simulink model "Wall_Model_Version_1_5_2016a"  (R2017b)
settings: Solver=ode3  StartTime=0.0  StopTime=1000  FixedStep=Ts  RelTol=1e-3  EnableMultiTasking=on
InitFcn:
  | clc;
  | clear all;
  | close all;
  | Ts=1
  | Duration=36000;
  | %% Coefficients of Rs and Cs
  | 
  | %% Front Wall
  | l1 = 7.37;
  | b1 = 2.63;
  | y1 = 0.5;
  | x1 = 0.33;
  | y2 = 0.5;
  | x2 = 0.33;
  | x3 = 0.33;
  | 
  | %% Left Wall
  | l2 = 10.11;
  | b2 = 2.63;
  | y3 = 0.5;
  | x4 = 0.33;
  | y4 = 0.5;
  | x5 = 0.33;
  | x6 = 0.33;
  | 
  | %% Left Wall Glass
  | x4_g = 0.5;
  | x5_g = 0.5;
  | y3_g = 1;
  | 
  | %% Right Wall
  | l3 = 7.37;
  | b3 = 2.63;
  | y5 = 0.5;
  | x7 = 0.33;
  | y6 = 0.5;
  | x8 = 0.33;
  | x9 = 0.33;
  | 
  | %% Back Wall
  | l4 = 10.11;
  | b4 = 2.63;
  | y7 = 1;
  | x10 = 0.5;
  | %y8 = 0.5;
  | x11 = 0.5;
  | %x12= 0.33;
  | 
  | %% Roof
  | l5 = 10.11;
  | b5 = 7.37;
  | y9 = 0.5;
  | x13 = 0.33;
  | y10 = 0.5;
  | x14 = 0.33;
  | x15 = 0.33;
  | 
  | %% Floor
  | l6 = 10.11;
  | b6 = 7.37;
  | y11 = 0.5;
  | x16 = 0.33;
  | y12 = 0.5;
  | x17 = 0.33;
  | x18 = 0.33;
  | 
  | %%Areas
  | A1 = l1 * b1;
  | A2 = l2 * b2;
  | A3 = l3 * b3;
  | A4 = l4 * b4;
  | A5 = l5 * b5;
  | A6 = l6 * b6;
  | 
  | %% Initial Temperatures at the surfaces
  | T1_initial_front=301;
  | T2_initial_front=300;
  | 
  | T1_initial_left=301;
  | T2_initial_left=300;
  | 
  | T1_initial_right=301;
  | T2_initial_right=300;
  | 
  | T1_initial_back=301;
  | T2_initial_back=300;
  | 
  | T1_initial_roof=301;
  | T2_initial_roof=300;
  | 
  | T1_initial_floor=301;
  | T2_initial_floor=300;
  | 
  | ri = 0.1300; % m2 K/W resistance of inner surface of brick wall
  | rso = 0.04; % m2 K/W resistance of outer surface of the wall
  | 
  | %% Density of Building materials in the room
  | p_conc    = 1700; % kg/m3 density of concrete
  | p_pstr     = 1000; % kg/m3 density of plastering
  | p_gb       = 1100; % kg/m3 density of gypsum board
  | p_glass    = 2500; % kg/m3 density of glass
  | p_swood  = 550;   % kg/m3 density of soft-wood
  | 
  | %% Thermal heat capacity of the building materials in the room
  | c_conc    = 840;  % J/kg K heat capacity of concrete
  | c_pstr     = 1000;  %J/kg K heat capacity of plastering
  | c_gb       = 1090; % J/kg K heat capacity of gypsum board
  | c_glass    = 840;  % J/kg K heat capacity of glass
  | c_swood  = 1700; % J/kg K heat capacity of soft-wood
  | 
  | %% Thermal conductivity(lamda) of building materials in the room
  | l_conc    = 0.8;  % W/m K Thermal conductivity of concrete
  | l_pstr     = 0.013;  % W/m K Thermal conductivity of plastering
  | l_gb       = 0.35; % W/m K Thermal conductivity of gypsum board
  | l_glass    = 0.8;  % W/m K Thermal conductivity of glass
  | l_swood  = 0.08; % W/m K Thermal conductivity of soft-wood
  | 
  | %% Standard thickness of materials used
  | d_conc = 0.01;  % m Thickness of concrete BCA standard
  | d_pstr = 0.005; % m Thickness of plastering BCA standard
  | d_glass = 0.015; % m Thickness of glass wall widely used
  | d_swood = 0.01; % m Thickness of softwood on the right wall
  | d_gb = 0.015; % m Thickness of gypsum board
  | 
  | %% Resistance and Capacitance of front Wall
  | Rth1 =( ri + rso + (d_conc/l_conc) + (d_pstr/l_pstr))/(A1); % Thermal resistance
  | Cth1 = A1*(d_conc*p_conc*c_conc + d_pstr*p_pstr*c_pstr) ; % Thermal Capacitance
  | 
  | %% Resistance and Capacitance of left Wall concrete
  | A_conc = A2 * 0.5; % Half of the wall on the left is  glass wall
  | Rth2 =( ri + rso + (d_conc/l_conc) + (d_pstr/l_pstr))/(A_conc); % Thermal resistance
  | Cth2 = A_conc*(d_conc*p_conc*c_conc + d_pstr*p_pstr*c_pstr); % Thermal Capacitance
  | 
  | %% Resistance and Capacitance of left Wall glass
  | A_glass = A2 * 0.5; % Half of the wall on the left is  glass wall
  | Rth2_g =(d_glass/l_glass) /(A_glass); % Thermal resistance
  | Cth2_g = A_glass*(d_glass*p_glass*c_glass ); % Thermal Capacitance
  | 
  | %% Resistance and Capacitance of right Wall
  | Rth3 = ( ri + rso+ (d_conc/l_conc) + (d_swood/l_swood))/(A3);% Thermal resistance
  | Cth3 = A3*(d_swood*p_swood*c_swood + d_conc*p_conc*c_conc ); % Thermal Capacitance
  | 
  | %% Resistance and Capacitance of back Wall
  | Rth4 =(d_glass/l_glass) /(A4); % Thermal resistance
  | Cth4 = A4*(d_glass*p_glass*c_glass ); % Thermal Capacitance
  | 
  | %% Resistance and Capacitance of roof Wall
  | Rth5 = (d_gb/l_gb)/(A5);% Thermal resistance
  | Cth5 = A5*(d_gb*p_gb*c_gb ); % Thermal Capacitance
  | 
  | %% Resistance and Capacitance of floor Wall
  | Rth6 = (d_gb/l_gb)/(A6);% Thermal resistance
  | Cth6 = A6*(d_gb*p_gb*c_gb ); % Thermal Capacitance
  | 
  | %% Volume and mass of room
  | density_of_air = 1.184; % kg/m3 at 25 deg. K
  | volume = l1*l2*b1; % m3
  | mass = volume * density_of_air ;% kg
  | specific_heat = 1.005; % J/kg deg.K
  | tic;
libraries: powerlib x69, simulink x1
settings Model: Creator=elekkr  LastModifiedBy=e0154145
settings DataIOCC: LimitDataPoints=on  SaveFormat=Array
settings OptimizationCC: LifeSpan=inf
settings DebuggingCC: UnconnectedInputMsg=none  UnconnectedOutputMsg=none  UnconnectedLineMsg=none  SFUnexpectedBacktrackingDiag=warning  SFNoUnconditionalDefaultTransitionDiag=warning  SFExecutionAtInitializationDiag=none
settings HardwareCC: ProdBitPerPointer=32  ProdBitPerSizeT=32  ProdBitPerPtrDiffT=32  ProdLargestAtomicFloat=None  ProdIntDivRoundTo=Undefined  ProdEndianess=Unspecified  ProdWordSize=32  ProdHWDeviceType=32-bit Generic
settings ModelReferenceCC: PropagateSignalLabelsOutOfModel=off
settings CodeAppCC: StateflowObjectComments=on
settings GRTTargetCC: TargetLangStandard=C89/C90 (ANSI)  GeneratePreprocessorConditionals=Disable all
settings ConfigComp: CovMetricSettings=dw  CovHtmlReporting=on  CovSaveCumulativeToWorkspaceVar=on  CovSaveSingleToWorkspaceVar=on  CovExternalEMLEnable=off
settings SimscapeCC: SimscapeNormalizeSystem=off

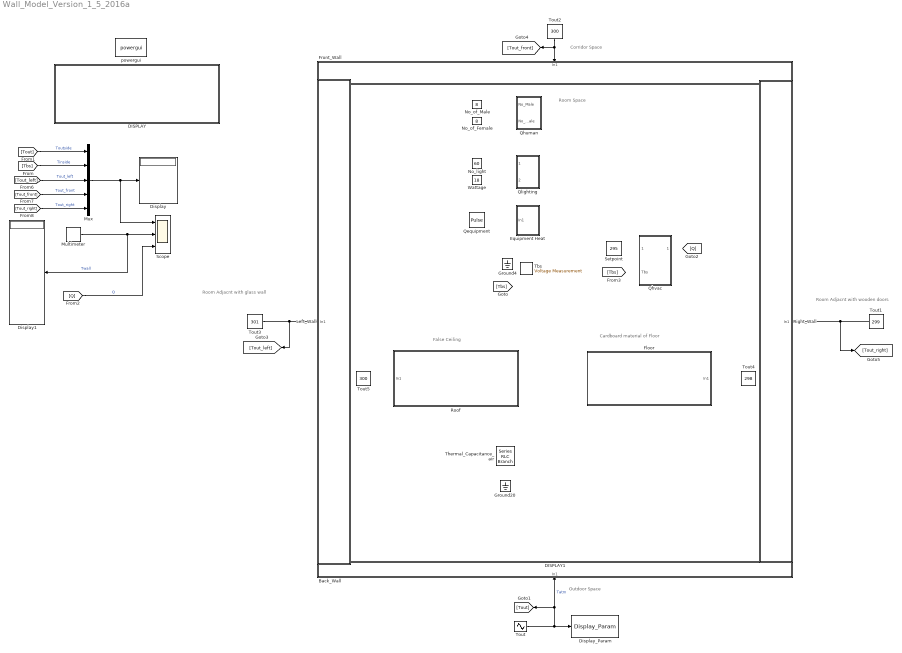
== system Wall_Model_Version_1_5_2016a ==
  note: False Ceiling
  note: Cardboard material of Floor
  note: Room Adjacnt with wooden doors
  note: Corridor Space
  note: Room Adjacnt with glass wall
  note: Outdoor Space
  note: Room Space
  Back_Wall : Subsystem
      mask Display: fprintf('Temperature Outside= 303 deg. K\n')
  DISPLAY : Subsystem  mask(GBIC - Simulation Speed){}
      settings: AttributesFormatString=22.03
      mask Display: fprintf('Simulation_Time_Elapsed=1000.00 seconds\nPhysical_Time_Elapsed=22.03 seconds\nSimulation_Speed=45.39 times')
  DISPLAY1 : Subsystem  mask(GBIC - Simulation Speed){}
      settings: AttributesFormatString=35.01
  Display : Display
  Display1 : Display
  Display_Param : M-S-Function  FunctionName=Display_Param
  Equipment Heat : Subsystem
  Floor : Subsystem
      mask Display: fprintf('Temperature \n Below= \n298 deg. K\n')
  Front_Wall : Subsystem
      mask Display: fprintf('Temperature Corridor= 300 deg. K\n')
  Ground20 : powerlib/Elements/Ground  LConnTagsString=a
  Ground4 : powerlib/Elements/Ground  LConnTagsString=a
  Left_Wall : Subsystem
      mask Display: fprintf('Temperature \n Left Room= \n301 deg. K\n')
  Multimeter : powerlib/Measurements/Multimeter  PhasorSimulation=off  OutputType=Complex  sel=[1 2 3 4 5 6 7 8 10 11 12 13]  L=13  Gain=[1 1 1 1 1 1 1 1 1 1 1 1]  yselected={'Ub: Back_Wall/y7*Cth4','Ub: Floor/y11*Cth6','Ub: Floor/y12*Cth6','Ub: Front_Wall/y1*Cth1','Ub: Front_Wall/y2*Cth1','Ub: Left_Wall/y3*Cth2','Ub: Left_Wall/y3_g*Cth2_g','Ub: Left_Wall/y4*Cth2','Ub: Right_Wall/y5*Cth3','Ub: Right_Wall/y6*Cth3','Ub: Roof/y10*Cth5','Ub: Roof/y9*Cth5'};  PSBOutputType=1  PSBequivalent=0  AxesSetting=[0,0.1,-100,100]  Display=0  SavedBlockNames=-11
  Mux : Mux  Inputs=5
  No_light : Constant  Value=60
  No_of_Female : Constant  Value=8
  No_of_Male : Constant  Value=8
  Qequipment : DiscretePulseGenerator  PulseType=Time based  Amplitude=3200  Period=1e8  PulseWidth=50
  Qhuman : Subsystem
  Qhvac : Subsystem
  Qlighting : Subsystem
  Right_Wall : Subsystem
      mask Display: fprintf('Temperature \n Right Room= \n299 deg. K\n')
  Roof : Subsystem
      mask Display: fprintf('Temperature \n Above Roof= \n300 deg. K\n')
  Scope : Scope  NumInputPorts=3
  Setpoint : Constant  Value=295
  Tbs : powerlib/Measurements/Voltage Measurement  PhasorSimulation=off  OutputType=Magnitude  PSBequivalent=0
  Thermal_Capacitance_air : powerlib/Elements/Series RLC Branch  LConnTagsString=__new0  RConnTagsString=__new0  BranchType=C  Resistance=0  Inductance=1e-3  SetiL0=off  InitialCurrent=0  Capacitance=density_of_air * volume * specific_heat  Setx0=on  InitialVoltage=298  Measurements=Branch voltage
  Tout : Sin  Amplitude=5  Bias=303  Frequency=2*pi/(12*3600)  SampleTime=0
  Tout1 : Constant  Value=299
  Tout2 : Constant  Value=300
  Tout3 : Constant  Value=301
  Tout4 : Constant  Value=298
  Tout5 : Constant  Value=300
  Wattage : Constant  Value=18
  powergui : powerlib/powergui  Priority=1  SimulationMode=Discrete  SampleTime=Ts  frequency=60  Iterations=50  frequencyindice=0  Pbase=100e6  ErrMax=1e-4  UnitsV=kV  UnitsW=MW  buscounter=0  FunctionMessages=off  echomessages=off  EnableUseOfTLC=off  CurrentSourceSwitches=off  DisableSnubberDevices=off  DisableRonSwitches=off  DisableVfSwitches=off  DisplayEquations=off  SolverType=Tustin/Backward Euler (TBE)  Interpol=off  ExternalGateDelay=off  methode=off  Ts=100  x0status=blocks  SPID=off  SwTol=0  HookPort=off  RestoreLinks=warning  ResistiveCurrentMeasurement=off  Frange=[0:2:500]  Ylog=off  Xlog=on  ShowGrid=off  save=off  variable=ZData  structure=0  ZoomFFT=off  StartTime=0.0  cycles=1  DisplayStyle=1  fundamental=60  FreqAxis=off  MaxFrequency=1000  frequencyindicesteady=1  RmsSteady=1  display=off
  wires:
  Mux/1 -> Scope/1, Display/1
  [Tbs] -> Mux/2  "Tinside"
  [Tout] -> Mux/1  "Toutside"
  Multimeter/1 -> Display1/1, Scope/2  "Twall"
  [Q] -> Scope/3  "Q"
  Tbs/1 -> [Tbs]
  Tout/1 -> Display_Param/1, Back_Wall/1(In1), [Tout]  "Tatm"
  Qequipment/1 -> Equipment Heat/1(In1)
  Tout1/1 -> [Tout_right], Right_Wall/1(In1)
  Tout4/1 -> Floor/1(In1)
  Tout5/1 -> Roof/1(In1)
  Tout2/1 -> [Tout_front], Front_Wall/1(In1)
  Tout3/1 -> [Tout_left], Left_Wall/1(In1)
  [Tout_left] -> Mux/3  "Tout_left"
  [Tout_right] -> Mux/5  "Tout_right"
  [Tout_front] -> Mux/4  "Tout_front"
  No_light/1 -> Qlighting/1("No_light ")
  Wattage/1 -> Qlighting/2(Wattage)
  No_of_Male/1 -> Qhuman/1("No_Male ")
  No_of_Female/1 -> Qhuman/2(No_Female)
  Setpoint/1 -> Qhvac/1(Setpoint)
  [Tbs] -> Qhvac/2(Tbs)
  Qhvac/1(Qhvac) -> [Q]
  connections:
  Equipment Heat/RConn1 -- Qhvac/RConn1 -- Right_Wall/RConn1 -- Thermal_Capacitance_air/LConn1 -- Back_Wall/RConn1 -- Floor/RConn1 -- Roof/RConn1 -- Left_Wall/RConn1 -- Tbs/LConn1 -- Qlighting/RConn1 -- Qhuman/RConn1 -- Front_Wall/RConn1
  Ground4/LConn1 -- Tbs/LConn2
  Ground20/LConn1 -- Thermal_Capacitance_air/RConn1

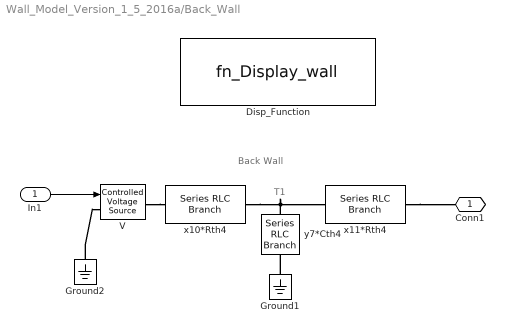
== system Wall_Model_Version_1_5_2016a/Back_Wall ==
  note: T1
  note: Back Wall
  In1 : Inport
  Disp_Function : M-S-Function  FunctionName=fn_Display_wall
  Ground1 : powerlib/Elements/Ground  LConnTagsString=a
  Ground2 : powerlib/Elements/Ground  LConnTagsString=a
  V : powerlib/Electrical Sources/Controlled Voltage Source  Initialize=on  Source_Type=AC  Amplitude=0  Phase=0  Frequency=0  Measurements=None
  x10*Rth4 : powerlib/Elements/Series RLC Branch  LConnTagsString=__new0  RConnTagsString=__new0  BranchType=R  Resistance=x10*Rth4  Inductance=1e-3  SetiL0=off  InitialCurrent=0  Capacitance=1e-6  Setx0=off  InitialVoltage=0  Measurements=None
  x11*Rth4 : powerlib/Elements/Series RLC Branch  LConnTagsString=__new0  RConnTagsString=__new0  BranchType=R  Resistance=x11*Rth4  Inductance=1e-3  SetiL0=off  InitialCurrent=0  Capacitance=1e-6  Setx0=off  InitialVoltage=0  Measurements=None
  y7*Cth4 : powerlib/Elements/Series RLC Branch  LConnTagsString=__new0  RConnTagsString=__new0  BranchType=C  Resistance=0  Inductance=1e-3  SetiL0=off  InitialCurrent=0  Capacitance=y7*Cth4  Setx0=on  InitialVoltage=T1_initial_back  Measurements=Branch voltage
  Conn1 : PMIOPort  Side=Right
  wires:
  In1/1 -> V/1
  connections:
  Ground2/LConn1 -- V/LConn1
  V/RConn1 -- x10*Rth4/LConn1
  x10*Rth4/RConn1 -- y7*Cth4/LConn1 -- x11*Rth4/LConn1
  Ground1/LConn1 -- y7*Cth4/RConn1
  x11*Rth4/RConn1 -- Conn1/RConn1

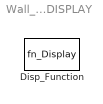
== system Wall_Model_Version_1_5_2016a/DISPLAY ==
  Disp_Function : M-S-Function  FunctionName=fn_Display

== system Wall_Model_Version_1_5_2016a/DISPLAY1 ==
  Disp_Function : M-S-Function  FunctionName=fn_Display_Room

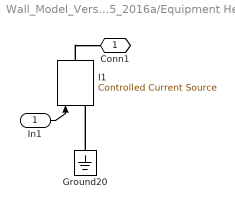
== system Wall_Model_Version_1_5_2016a/Equipment Heat ==
  In1 : Inport
  Ground20 : powerlib/Elements/Ground  LConnTagsString=a
  I1 : powerlib/Electrical Sources/Controlled Current Source  Initialize=off  Source_Type=AC  Amplitude=1  Phase=0  Frequency=0  Measurements=None
  Conn1 : PMIOPort  Side=Right
  wires:
  In1/1 -> I1/1
  connections:
  Ground20/LConn1 -- I1/LConn1
  I1/RConn1 -- Conn1/RConn1

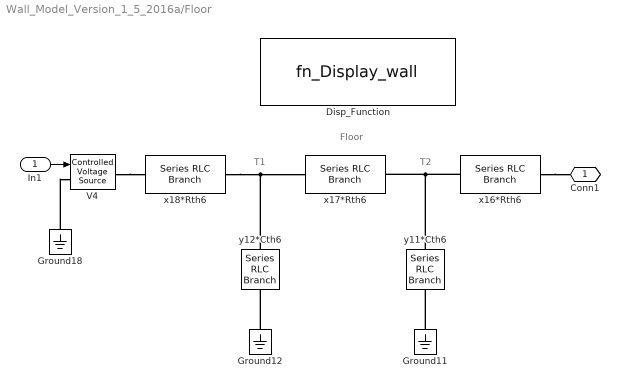
== system Wall_Model_Version_1_5_2016a/Floor ==
  note: T2
  note: T1
  note: Floor
  In1 : Inport
  Disp_Function : M-S-Function  FunctionName=fn_Display_wall
  Ground11 : powerlib/Elements/Ground  LConnTagsString=a
  Ground12 : powerlib/Elements/Ground  LConnTagsString=a
  Ground18 : powerlib/Elements/Ground  LConnTagsString=a
  V4 : powerlib/Electrical Sources/Controlled Voltage Source  Initialize=on  Source_Type=AC  Amplitude=0  Phase=0  Frequency=0  Measurements=None
  x16*Rth6 : powerlib/Elements/Series RLC Branch  LConnTagsString=__new0  RConnTagsString=__new0  BranchType=R  Resistance=x16*Rth6  Inductance=1e-3  SetiL0=off  InitialCurrent=0  Capacitance=1e-6  Setx0=off  InitialVoltage=0  Measurements=None
  x17*Rth6 : powerlib/Elements/Series RLC Branch  LConnTagsString=__new0  RConnTagsString=__new0  BranchType=R  Resistance=x17*Rth6  Inductance=1e-3  SetiL0=off  InitialCurrent=0  Capacitance=1e-6  Setx0=off  InitialVoltage=0  Measurements=None
  x18*Rth6 : powerlib/Elements/Series RLC Branch  LConnTagsString=__new0  RConnTagsString=__new0  BranchType=R  Resistance=x18*Rth6  Inductance=1e-3  SetiL0=off  InitialCurrent=0  Capacitance=1e-6  Setx0=off  InitialVoltage=0  Measurements=None
  y11*Cth6 : powerlib/Elements/Series RLC Branch  LConnTagsString=__new0  RConnTagsString=__new0  BranchType=C  Resistance=0  Inductance=1e-3  SetiL0=off  InitialCurrent=0  Capacitance=y11*Cth6  Setx0=on  InitialVoltage=T1_initial_floor  Measurements=Branch voltage
  y12*Cth6 : powerlib/Elements/Series RLC Branch  LConnTagsString=__new0  RConnTagsString=__new0  BranchType=C  Resistance=0  Inductance=1e-3  SetiL0=off  InitialCurrent=0  Capacitance=y12*Cth6  Setx0=on  InitialVoltage=T2_initial_floor  Measurements=Branch voltage
  Conn1 : PMIOPort  Side=Right
  wires:
  In1/1 -> V4/1
  connections:
  V4/RConn1 -- x18*Rth6/LConn1
  y11*Cth6/LConn1 -- x16*Rth6/LConn1 -- x17*Rth6/RConn1
  y12*Cth6/LConn1 -- x18*Rth6/RConn1 -- x17*Rth6/LConn1
  Ground18/LConn1 -- V4/LConn1
  Ground11/LConn1 -- y11*Cth6/RConn1
  Ground12/LConn1 -- y12*Cth6/RConn1
  x16*Rth6/RConn1 -- Conn1/RConn1

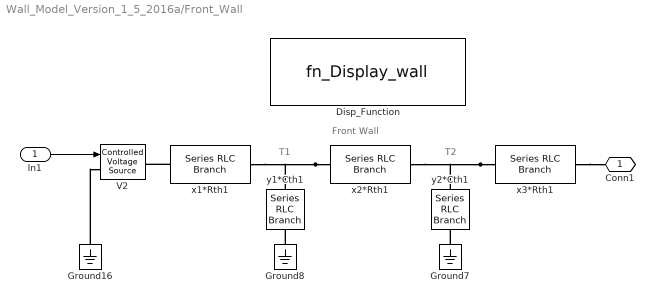
== system Wall_Model_Version_1_5_2016a/Front_Wall ==
  note: Front Wall
  note: T2
  note: T1
  In1 : Inport
  Disp_Function : M-S-Function  FunctionName=fn_Display_wall
  Ground16 : powerlib/Elements/Ground  LConnTagsString=a
  Ground7 : powerlib/Elements/Ground  LConnTagsString=a
  Ground8 : powerlib/Elements/Ground  LConnTagsString=a
  V2 : powerlib/Electrical Sources/Controlled Voltage Source  Initialize=on  Source_Type=AC  Amplitude=0  Phase=0  Frequency=0  Measurements=None
  x1*Rth1 : powerlib/Elements/Series RLC Branch  LConnTagsString=__new0  RConnTagsString=__new0  BranchType=R  Resistance=x1*Rth1  Inductance=1e-3  SetiL0=off  InitialCurrent=0  Capacitance=1e-6  Setx0=off  InitialVoltage=0  Measurements=None
  x2*Rth1 : powerlib/Elements/Series RLC Branch  LConnTagsString=__new0  RConnTagsString=__new0  BranchType=R  Resistance=x2*Rth1  Inductance=1e-3  SetiL0=off  InitialCurrent=0  Capacitance=1e-6  Setx0=off  InitialVoltage=0  Measurements=None
  x3*Rth1 : powerlib/Elements/Series RLC Branch  LConnTagsString=__new0  RConnTagsString=__new0  BranchType=R  Resistance=x3*Rth1  Inductance=1e-3  SetiL0=off  InitialCurrent=0  Capacitance=1e-6  Setx0=off  InitialVoltage=0  Measurements=None
  y1*Cth1 : powerlib/Elements/Series RLC Branch  LConnTagsString=__new0  RConnTagsString=__new0  BranchType=C  Resistance=0  Inductance=1e-3  SetiL0=off  InitialCurrent=0  Capacitance=y1*Cth1  Setx0=on  InitialVoltage=T1_initial_front  Measurements=Branch voltage
  y2*Cth1 : powerlib/Elements/Series RLC Branch  LConnTagsString=__new0  RConnTagsString=__new0  BranchType=C  Resistance=0  Inductance=1e-3  SetiL0=off  InitialCurrent=0  Capacitance=y2*Cth1  Setx0=on  InitialVoltage=T2_initial_front  Measurements=Branch voltage
  Conn1 : PMIOPort  Side=Right
  wires:
  In1/1 -> V2/1
  connections:
  Ground7/LConn1 -- y2*Cth1/RConn1
  x2*Rth1/LConn1 -- x1*Rth1/RConn1 -- y1*Cth1/LConn1
  x3*Rth1/LConn1 -- x2*Rth1/RConn1 -- y2*Cth1/LConn1
  Ground16/LConn1 -- V2/LConn1
  Ground8/LConn1 -- y1*Cth1/RConn1
  x1*Rth1/LConn1 -- V2/RConn1
  x3*Rth1/RConn1 -- Conn1/RConn1

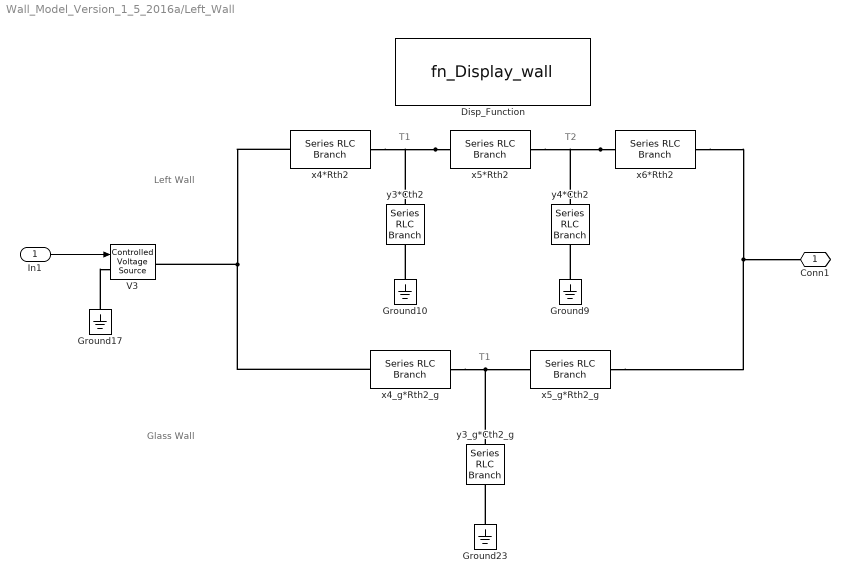
== system Wall_Model_Version_1_5_2016a/Left_Wall ==
  note: T1
  note: Glass Wall
  note: Left Wall
  note: T2
  note: T1
  In1 : Inport
  Disp_Function : M-S-Function  FunctionName=fn_Display_wall
  Ground{9..10,17,23} (4 alike) : powerlib/Elements/Ground  LConnTagsString=a
  V3 : powerlib/Electrical Sources/Controlled Voltage Source  Initialize=on  Source_Type=AC  Amplitude=0  Phase=0  Frequency=0  Measurements=None
  x4*Rth2 : powerlib/Elements/Series RLC Branch  LConnTagsString=__new0  RConnTagsString=__new0  BranchType=R  Resistance=x4*Rth2  Inductance=1e-3  SetiL0=off  InitialCurrent=0  Capacitance=1e-6  Setx0=off  InitialVoltage=0  Measurements=None
  x4_g*Rth2_g : powerlib/Elements/Series RLC Branch  LConnTagsString=__new0  RConnTagsString=__new0  BranchType=R  Resistance=x4_g*Rth2_g  Inductance=1e-3  SetiL0=off  InitialCurrent=0  Capacitance=1e-6  Setx0=off  InitialVoltage=0  Measurements=None
  x5*Rth2 : powerlib/Elements/Series RLC Branch  LConnTagsString=__new0  RConnTagsString=__new0  BranchType=R  Resistance=x5*Rth2  Inductance=1e-3  SetiL0=off  InitialCurrent=0  Capacitance=1e-6  Setx0=off  InitialVoltage=0  Measurements=None
  x5_g*Rth2_g : powerlib/Elements/Series RLC Branch  LConnTagsString=__new0  RConnTagsString=__new0  BranchType=R  Resistance=x5_g*Rth2_g  Inductance=1e-3  SetiL0=off  InitialCurrent=0  Capacitance=1e-6  Setx0=off  InitialVoltage=0  Measurements=None
  x6*Rth2 : powerlib/Elements/Series RLC Branch  LConnTagsString=__new0  RConnTagsString=__new0  BranchType=R  Resistance=x6*Rth2  Inductance=1e-3  SetiL0=off  InitialCurrent=0  Capacitance=1e-6  Setx0=off  InitialVoltage=0  Measurements=None
  y3*Cth2 : powerlib/Elements/Series RLC Branch  LConnTagsString=__new0  RConnTagsString=__new0  BranchType=C  Resistance=0  Inductance=1e-3  SetiL0=off  InitialCurrent=0  Capacitance=y3*Cth2  Setx0=on  InitialVoltage=T1_initial_left  Measurements=Branch voltage
  y3_g*Cth2_g : powerlib/Elements/Series RLC Branch  LConnTagsString=__new0  RConnTagsString=__new0  BranchType=C  Resistance=0  Inductance=1e-3  SetiL0=off  InitialCurrent=0  Capacitance=y3_g*Cth2_g  Setx0=on  InitialVoltage=T1_initial_left  Measurements=Branch voltage
  y4*Cth2 : powerlib/Elements/Series RLC Branch  LConnTagsString=__new0  RConnTagsString=__new0  BranchType=C  Resistance=0  Inductance=1e-3  SetiL0=off  InitialCurrent=0  Capacitance=y4*Cth2  Setx0=on  InitialVoltage=T2_initial_left  Measurements=Branch voltage
  Conn1 : PMIOPort  Side=Right
  wires:
  In1/1 -> V3/1
  connections:
  x5*Rth2/LConn1 -- x4*Rth2/RConn1 -- y3*Cth2/LConn1
  x6*Rth2/LConn1 -- x5*Rth2/RConn1 -- y4*Cth2/LConn1
  x4*Rth2/LConn1 -- x4_g*Rth2_g/LConn1 -- V3/RConn1
  x6*Rth2/RConn1 -- x5_g*Rth2_g/RConn1 -- Conn1/RConn1
  Ground10/LConn1 -- y3*Cth2/RConn1
  y3_g*Cth2_g/LConn1 -- x4_g*Rth2_g/RConn1 -- x5_g*Rth2_g/LConn1
  Ground23/LConn1 -- y3_g*Cth2_g/RConn1
  Ground9/LConn1 -- y4*Cth2/RConn1
  Ground17/LConn1 -- V3/LConn1

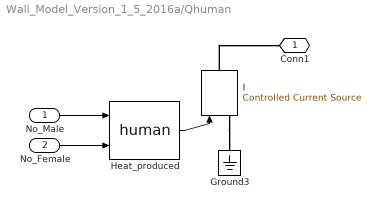
== system Wall_Model_Version_1_5_2016a/Qhuman ==
  "No_Male " : Inport
  No_Female : Inport  Port=2
  Ground3 : powerlib/Elements/Ground  LConnTagsString=a
  Heat_produced : M-S-Function  FunctionName=human
  I : powerlib/Electrical Sources/Controlled Current Source  Initialize=on  Source_Type=AC  Amplitude=1  Phase=0  Frequency=0  Measurements=None
  Conn1 : PMIOPort  Side=Right
  wires:
  "No_Male "/1 -> Heat_produced/1
  Heat_produced/1 -> I/1
  No_Female/1 -> Heat_produced/2
  connections:
  I/LConn1 -- Ground3/LConn1
  I/RConn1 -- Conn1/RConn1

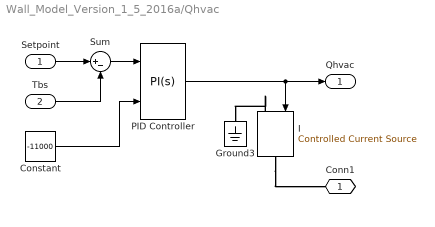
== system Wall_Model_Version_1_5_2016a/Qhvac ==
  Setpoint : Inport
  Tbs : Inport  Port=2
  Constant : Constant  Value=-11000
  Ground3 : powerlib/Elements/Ground  LConnTagsString=a
  I : powerlib/Electrical Sources/Controlled Current Source  Initialize=on  Source_Type=DC  Amplitude=5000  Phase=0  Frequency=0  Measurements=None
  PID Controller : simulink/Continuous/PID Controller  Controller=PI  TimeDomain=Continuous-time  SampleTime=-1  IntegratorMethod=Backward Euler  FilterMethod=Forward Euler  Form=Parallel  UseFilter=on  ControllerParametersSource=internal  P=73.2267691455224  I=36.1989767443259  D=-23089.3147185246  N=0.114288574843554  InitialConditionSource=external  InitialConditionForIntegrator=22  InitialConditionForFilter=0  ExternalReset=none  LimitOutput=off  UpperSaturationLimit=0  LowerSaturationLimit=-11000  LinearizeAsGain=off  AntiWindupMode=none  Kb=1  TrackingMode=off  Kt=1  PParamMin=[]  PParamMax=[]  IParamMin=[]  IParamMax=[]  DParamMin=[]  DParamMax=[]  NParamMin=[]  NParamMax=[]  KbParamMin=[]  KbParamMax=[]  KtParamMin=[]  KtParamMax=[]  POutMin=[]  POutMax=[]  IOutMin=[]  IOutMax=[]  DOutMin=[]  DOutMax=[]  NOutMin=[]  NOutMax=[]  KbOutMin=[]  KbOutMax=[]  KtOutMin=[]  KtOutMax=[]  IntegratorOutMin=[]  IntegratorOutMax=[]  FilterOutMin=[]  FilterOutMax=[]  SumOutMin=[]  SumOutMax=[]  SumI1OutMin=[]  SumI1OutMax=[]  SumI2OutMin=[]  SumI2OutMax=[]  SumI3OutMin=[]  SumI3OutMax=[]  SumDOutMin=[]  SumDOutMax=[]  SaturationOutMin=[]  SaturationOutMax=[]  IntegratorContinuousStateAttributes=''  IntegratorStateMustResolveToSignalObject=off  IntegratorRTWStateStorageClass=Auto  FilterContinuousStateAttributes=''  FilterStateMustResolveToSignalObject=off  FilterRTWStateStorageClass=Auto  DifferentiatorICPrevScaledInput=0  DifferentiatorOutMin=[]  DifferentiatorOutMax=[]  FilterDiffOutCoefMin=[]  FilterDiffOutCoefMax=[]  SumDenOutMin=[]  SumDenOutMax=[]  SumNumOutMin=[]  SumNumOutMax=[]  ReciprocalOutMin=[]  ReciprocalOutMax=[]  DivideOutMin=[]  DivideOutMax=[]  TunerSelectOption=Transfer Function Based (PID Tuner App)
  Sum : Sum  Inputs=|+-
  Conn1 : PMIOPort  Side=Right
  Qhvac : Outport
  wires:
  PID Controller/1 -> I/1, Qhvac/1
  Setpoint/1 -> Sum/1
  Tbs/1 -> Sum/2
  Sum/1 -> PID Controller/1
  Constant/1 -> PID Controller/2
  connections:
  I/RConn1 -- Conn1/RConn1
  I/LConn1 -- Ground3/LConn1

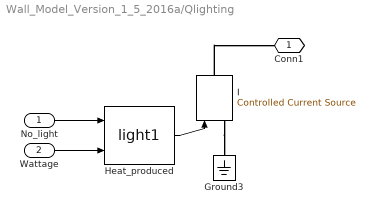
== system Wall_Model_Version_1_5_2016a/Qlighting ==
  "No_light " : Inport
  Wattage : Inport  Port=2
  Ground3 : powerlib/Elements/Ground  LConnTagsString=a
  Heat_produced : M-S-Function  FunctionName=light1
  I : powerlib/Electrical Sources/Controlled Current Source  Initialize=on  Source_Type=AC  Amplitude=1  Phase=0  Frequency=0  Measurements=None
  Conn1 : PMIOPort  Side=Right
  wires:
  "No_light "/1 -> Heat_produced/1
  Heat_produced/1 -> I/1
  Wattage/1 -> Heat_produced/2
  connections:
  I/LConn1 -- Ground3/LConn1
  I/RConn1 -- Conn1/RConn1

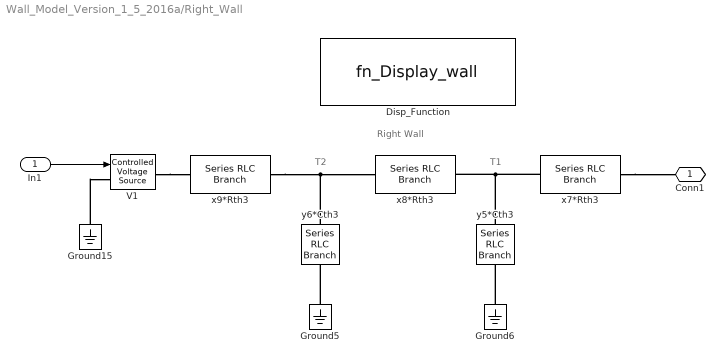
== system Wall_Model_Version_1_5_2016a/Right_Wall ==
  note: Right Wall
  note: T2
  note: T1
  In1 : Inport
  Disp_Function : M-S-Function  FunctionName=fn_Display_wall
  Ground15 : powerlib/Elements/Ground  LConnTagsString=a
  Ground5 : powerlib/Elements/Ground  LConnTagsString=a
  Ground6 : powerlib/Elements/Ground  LConnTagsString=a
  V1 : powerlib/Electrical Sources/Controlled Voltage Source  Initialize=on  Source_Type=AC  Amplitude=0  Phase=0  Frequency=0  Measurements=None
  x7*Rth3 : powerlib/Elements/Series RLC Branch  LConnTagsString=__new0  RConnTagsString=__new0  BranchType=R  Resistance=x7*Rth3  Inductance=1e-3  SetiL0=off  InitialCurrent=0  Capacitance=1e-6  Setx0=off  InitialVoltage=0  Measurements=None
  x8*Rth3 : powerlib/Elements/Series RLC Branch  LConnTagsString=__new0  RConnTagsString=__new0  BranchType=R  Resistance=x8*Rth3  Inductance=1e-3  SetiL0=off  InitialCurrent=0  Capacitance=1e-6  Setx0=off  InitialVoltage=0  Measurements=None
  x9*Rth3 : powerlib/Elements/Series RLC Branch  LConnTagsString=__new0  RConnTagsString=__new0  BranchType=R  Resistance=x9*Rth3  Inductance=1e-3  SetiL0=off  InitialCurrent=0  Capacitance=1e-6  Setx0=off  InitialVoltage=0  Measurements=None
  y5*Cth3 : powerlib/Elements/Series RLC Branch  LConnTagsString=__new0  RConnTagsString=__new0  BranchType=C  Resistance=0  Inductance=1e-3  SetiL0=off  InitialCurrent=0  Capacitance=y5*Cth3  Setx0=on  InitialVoltage=T1_initial_right  Measurements=Branch voltage
  y6*Cth3 : powerlib/Elements/Series RLC Branch  LConnTagsString=__new0  RConnTagsString=__new0  BranchType=C  Resistance=0  Inductance=1e-3  SetiL0=off  InitialCurrent=0  Capacitance=y6*Cth3  Setx0=on  InitialVoltage=T2_initial_right  Measurements=Branch voltage
  Conn1 : PMIOPort  Side=Right
  wires:
  In1/1 -> V1/1
  connections:
  x7*Rth3/RConn1 -- Conn1/RConn1
  x7*Rth3/LConn1 -- y5*Cth3/LConn1 -- x8*Rth3/RConn1
  y6*Cth3/LConn1 -- x9*Rth3/RConn1 -- x8*Rth3/LConn1
  Ground15/LConn1 -- V1/LConn1
  Ground5/LConn1 -- y6*Cth3/RConn1
  Ground6/LConn1 -- y5*Cth3/RConn1
  V1/RConn1 -- x9*Rth3/LConn1

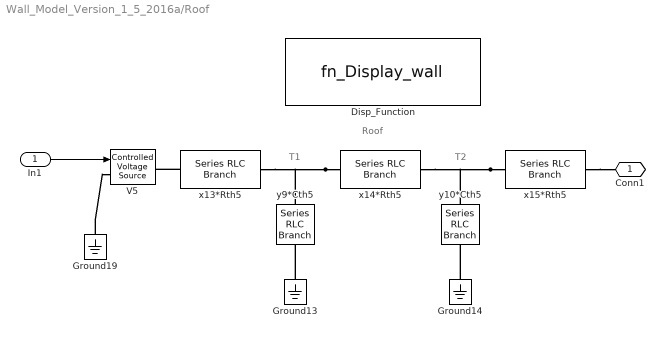
== system Wall_Model_Version_1_5_2016a/Roof ==
  note: T1
  note: T2
  note: Roof
  In1 : Inport
  Disp_Function : M-S-Function  FunctionName=fn_Display_wall
  Ground13 : powerlib/Elements/Ground  LConnTagsString=a
  Ground14 : powerlib/Elements/Ground  LConnTagsString=a
  Ground19 : powerlib/Elements/Ground  LConnTagsString=a
  V5 : powerlib/Electrical Sources/Controlled Voltage Source  Initialize=on  Source_Type=AC  Amplitude=0  Phase=0  Frequency=0  Measurements=None
  x13*Rth5 : powerlib/Elements/Series RLC Branch  LConnTagsString=__new0  RConnTagsString=__new0  BranchType=R  Resistance=x13*Rth5  Inductance=1e-3  SetiL0=off  InitialCurrent=0  Capacitance=1e-6  Setx0=off  InitialVoltage=0  Measurements=None
  x14*Rth5 : powerlib/Elements/Series RLC Branch  LConnTagsString=__new0  RConnTagsString=__new0  BranchType=R  Resistance=x14*Rth5  Inductance=1e-3  SetiL0=off  InitialCurrent=0  Capacitance=1e-6  Setx0=off  InitialVoltage=0  Measurements=None
  x15*Rth5 : powerlib/Elements/Series RLC Branch  LConnTagsString=__new0  RConnTagsString=__new0  BranchType=R  Resistance=x15*Rth5  Inductance=1e-3  SetiL0=off  InitialCurrent=0  Capacitance=1e-6  Setx0=off  InitialVoltage=0  Measurements=None
  y10*Cth5 : powerlib/Elements/Series RLC Branch  LConnTagsString=__new0  RConnTagsString=__new0  BranchType=C  Resistance=0  Inductance=1e-3  SetiL0=off  InitialCurrent=0  Capacitance=y10*Cth5  Setx0=on  InitialVoltage=T2_initial_roof  Measurements=Branch voltage
  y9*Cth5 : powerlib/Elements/Series RLC Branch  LConnTagsString=__new0  RConnTagsString=__new0  BranchType=C  Resistance=0  Inductance=1e-3  SetiL0=off  InitialCurrent=0  Capacitance=y9*Cth5  Setx0=on  InitialVoltage=T1_initial_roof  Measurements=Branch voltage
  Conn1 : PMIOPort  Side=Right
  wires:
  In1/1 -> V5/1
  connections:
  Ground14/LConn1 -- y10*Cth5/RConn1
  x15*Rth5/RConn1 -- Conn1/RConn1
  x14*Rth5/LConn1 -- x13*Rth5/RConn1 -- y9*Cth5/LConn1
  x15*Rth5/LConn1 -- x14*Rth5/RConn1 -- y10*Cth5/LConn1
  Ground19/LConn1 -- V5/LConn1
  x13*Rth5/LConn1 -- V5/RConn1
  Ground13/LConn1 -- y9*Cth5/RConn1
